simulink model "motionsystem_control_simulation"  (R2017a)
settings: Solver=FixedStepAuto  StartTime=0.0  StopTime=30  FixedStep=dt  RelTol=1e-3
values from neighbouring files (symbols this model uses):
  dt = 0.567    [SimulinkMotionPlot.m]    (also in f.m = 0.001; fJacobian.m = 0.001; h.m = 0.001; hJacobian.m = 0.001)
  K = lqr(A,B,Q_LQR, R_LQR)    [initialize_controller_motionsystem.m]
  Ki = KI(:,1:Ni)    [initialize_controller_motionsystem.m]
  p_init = [2.6192; 0; 2.24]    [initialize_controller_motionsystem.m]
  p_t_init = zeros(3,1)    [initialize_controller_motionsystem.m]
  phi_init = [phix_init; phiy_init]    [initialize_controller_motionsystem.m]
  Pt_init = [-2.395; 3.811; -3.255]    [initialize_controller_motionsystem.m]
libraries: sharedTrackingLibrary x1
settings Model: Creator=Jan  LastModifiedBy=Jan

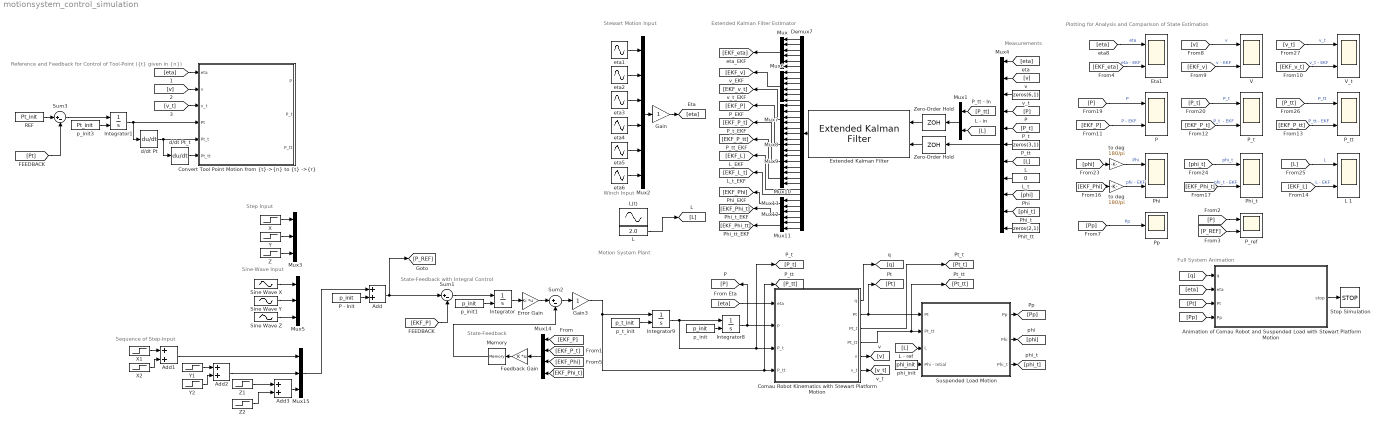
== system motionsystem_control_simulation ==
  note: Step Input
  note: Sine-Wave Input
  note: Sequence of Step-Input
  note: Motion System Plant
  note: Measurements
  note: State-Feedback
  note: Extended Kalman Filter Estimator
  note: Winch Input
  note: Full System Animation
  note: Stewart Motion Input
  note: Plotting for Analysis and Comparison of State Estimation
  note: State-Feedback with Integral Control
  note: Reference and Feedback for Control of Tool-Point
      | ({t} given in {n})
  " L_t " : Constant  Value=0
  " P_tt " : Constant  Value=zeros(3,1)
  " Phit_tt " : Constant  Value=zeros(2,1)
  " Zero-Order Hold " : ZeroOrderHold  SampleTime=dt
  " v_t " : Constant  Value=zeros(6,1)
  Add{,1..3} (4 alike) : Sum
  Animation of Comau Robot and Suspended Load with Stewart Platform Motion : MATLAB Function  TreatAsAtomicUnit=on  SystemSampleTime=0.1
  Comau Robot Kinematics with Stewart Platform Motion : Subsystem
  "Convert Tool Point Motion from {t}->{n} to {t} ->{r}" : MATLAB Function  TreatAsAtomicUnit=on
  Demux7 : Demux  Outputs=35
  Error Gain : Gain  Gain=Ki  Multiplication=Matrix(K*u)
  Eta1 : Scope  NumInputPorts=2
  Extended Kalman Filter : sharedTrackingLibrary/Extended Kalman Filter  StateTransitionFcn=f  HasStateTransitionJacobianFcn=on  StateTransitionJacobianFcn=fJacobian  HasAdditiveProcessNoise=Additive  ProcessNoise=Q_EKF  HasTimeVaryingProcessNoise=off  HasStateTransitionFcnExtraArgument=1  InitialState=EKF_init  InitialStateCovariance=P_EKF  MeasurementFcn1=h  HasMeasurementJacobianFcn1=on  MeasurementJacobianFcn1=hJacobian  HasMeasurementEnablePort1=off  HasAdditiveMeasurementNoise1=Additive  MeasurementNoise1=R_EKF  HasTimeVaryingMeasurementNoise1=off  HasMeasurementFcnExtraArgument1=0  MeasurementFcn2=myMeasurementFcn  HasMeasurementJacobianFcn2=off  HasMeasurementEnablePort2=off  HasAdditiveMeasurementNoise2=Additive  MeasurementNoise2=1  HasTimeVaryingMeasurementNoise2=off  HasMeasurementFcnExtraArgument2=0  MeasurementFcn3=myMeasurementFcn  HasMeasurementJacobianFcn3=off  HasMeasurementEnablePort3=off  HasAdditiveMeasurementNoise3=Additive  MeasurementNoise3=1  HasTimeVaryingMeasurementNoise3=off  HasMeasurementFcnExtraArgument3=0  MeasurementFcn4=myMeasurementFcn  HasMeasurementJacobianFcn4=off  HasMeasurementEnablePort4=off  HasAdditiveMeasurementNoise4=Additive  MeasurementNoise4=1  HasTimeVaryingMeasurementNoise4=off  HasMeasurementFcnExtraArgument4=0  MeasurementFcn5=myMeasurementFcn  HasMeasurementJacobianFcn5=off  HasMeasurementEnablePort5=off  HasAdditiveMeasurementNoise5=Additive  MeasurementNoise5=1  HasTimeVaryingMeasurementNoise5=off  HasMeasurementFcnExtraArgument5=0  EnableMultirate=off  StateTransitionFcnSampleTime=1  MeasurementFcn1SampleTime=1  MeasurementFcn2SampleTime=1  MeasurementFcn3SampleTime=1  MeasurementFcn4SampleTime=1  MeasurementFcn5SampleTime=1  UseCurrentEstimator=on  OutputStateCovariance=off  DataType=double  SampleTime=dt  NumberOfMeasurements=1
  Feedback Gain : Gain  Gain=K  Multiplication=Matrix(K*u)
  Gain : Gain
  Gain3 : Gain
  Integrator{,1,8..9} (4 alike) : Integrator  InitialConditionSource=external
  L : Constant  Value=2.0
  L 1 : Scope  NumInputPorts=2
  L(t) : Sin  Amplitude=0.75  Bias=2.0  Frequency=2*pi*0.05  SampleTime=0
  Memory : Memory
  Mux{,2,6..7} (4 alike) : Mux  Inputs=6
  Mux{1,11..13} (4 alike) : Mux  Inputs=2
  Mux{3,5,8..10,15} (6 alike) : Mux  Inputs=3
  Mux14 : Mux
  Mux4 : Mux  Inputs=11
  P : Scope  NumInputPorts=2
  P - Init : Constant  Value=p_init
  P_ref : Scope  NumInputPorts=2
  P_t : Scope  NumInputPorts=2
  P_tt : Scope  NumInputPorts=2
  Phi : Scope  NumInputPorts=2
  Phi_t : Scope  NumInputPorts=2
  "Pp   " : Scope
  REF : Constant  Value=Pt_init
  Sine Wave X : Sin  Amplitude=0.5  Frequency=2*pi*0.07  SampleTime=0
  Sine Wave Y : Sin  Amplitude=0.3  Frequency=2*pi*0.09  SampleTime=0
  Sine Wave Z : Sin  Amplitude=0.25  Frequency=2*pi*0.15  SampleTime=0
  Stop Simulation : Stop
  Sum1 : Sum  Inputs=|+-
  Sum2 : Sum  Inputs=|+-
  Sum3 : Sum  Inputs=|+-
  Suspended Load Motion : Subsystem
  V : Scope  NumInputPorts=2
  V_t : Scope  NumInputPorts=2
  X : Step  Time=0  After=0.4  SampleTime=0
  X1 : Step  After=0.4  SampleTime=0
  X2 : Step  Time=10  After=-0.8  SampleTime=0
  Y : Step  Time=0  After=0.4  SampleTime=0
  Y1 : Step  Time=2  After=0.4  SampleTime=0
  Y2 : Step  Time=13  After=-0.8  SampleTime=0
  Z : Step  Time=0  After=0.4  SampleTime=0
  Z1 : Step  Time=3  After=0.4  SampleTime=0
  Z2 : Step  Time=9  After=-0.2  SampleTime=0
  "Zero-Order Hold " : ZeroOrderHold  SampleTime=dt
  d/dt Pt : Derivative
  d/dt Pt_t : Derivative
  eta1 : Sin  Amplitude=0.1  Frequency=2*pi*0.1  Phase=0/180*pi  SampleTime=0
  eta2 : Sin  Amplitude=0.1  Frequency=2*pi*0.2  Phase=45/180*pi  SampleTime=0
  eta3 : Sin  Amplitude=0.2  Frequency=2*pi*0.1  Phase=90/180*pi  SampleTime=0
  eta4 : Sin  Amplitude=5/180*pi  Frequency=2*pi*0.1  Phase=0/180*pi  SampleTime=0
  eta5 : Sin  Amplitude=5/180*pi  Frequency=2*pi*0.15  Phase=90/180*pi  SampleTime=0
  eta6 : Sin  Amplitude=5/180*pi  Frequency=2*pi*0.2  Phase=120/180*pi  SampleTime=0
  "p_init " : Constant  Value=p_init
  p_init1 : Constant  Value=p_init
  p_init3 : Constant  Value=Pt_init
  p_t_init : Constant  Value=p_t_init
  phi_init : Constant  Value=phi_init
  to deg : Gain  Gain=180/pi
  "to deg    " : Gain  Gain=180/pi
  wires:
  Comau Robot Kinematics with Stewart Platform Motion/4(Pt_tt) -> [Pt_tt], Suspended Load Motion/2(Pt_tt)
  eta2/1 -> Mux2/2
  Mux2/1 -> Gain/1
  eta3/1 -> Mux2/3
  phi_init/1 -> Suspended Load Motion/4(Phi - Intial)
  eta1/1 -> Mux2/1
  eta6/1 -> Mux2/6
  eta5/1 -> Mux2/5
  Comau Robot Kinematics with Stewart Platform Motion/2(Pt) -> [Pt], Suspended Load Motion/1(Pt)
  eta4/1 -> Mux2/4
  Gain/1 -> [eta]
  Integrator8/1 -> [P], Comau Robot Kinematics with Stewart Platform Motion/2(P)
  "p_init "/1 -> Integrator8/2
  p_t_init/1 -> Integrator9/2
  Comau Robot Kinematics with Stewart Platform Motion/3(Pt_t) -> [Pt_t]
  Suspended Load Motion/3(Phi_t) -> [phi_t]
  Suspended Load Motion/2(Phi) -> [phi]
  Comau Robot Kinematics with Stewart Platform Motion/5(v) -> [v]
  Comau Robot Kinematics with Stewart Platform Motion/6(v_t) -> [v_t]
  Sum1/1 -> Integrator/1
  [EKF_P] -> Sum1/2
  Integrator/1 -> Error Gain/1
  Error Gain/1 -> Sum2/1
  Sum2/1 -> Gain3/1
  [P_tt] -> Mux1/1
  " Phit_tt "/1 -> Mux4/11
  Demux7/16 -> Mux7/4
  Demux7/14 -> Mux7/2
  Mux1/1 -> "Zero-Order Hold "/1
  [eta] -> Mux4/1
  Demux7/3 -> Mux/3
  Demux7/1 -> Mux/1
  [v] -> Mux4/2
  [L] -> Mux4/7
  Demux7/9 -> Mux6/3
  Demux7/4 -> Mux/4
  Demux7/13 -> Mux7/1
  Demux7/34 -> Mux11/1
  Demux7/19 -> Mux8/1
  Demux7/2 -> Mux/2
  Mux9/1 -> [EKF_P_t]
  Demux7/28 -> [EKF_L]
  [P] -> Mux4/4
  Mux13/1 -> [EKF_Phi]
  " P_tt "/1 -> Mux4/6
  Demux7/21 -> Mux8/3
  [P_t] -> Mux4/5
  Demux7/30 -> Mux13/1
  Demux7/22 -> Mux9/1
  " Zero-Order Hold "/1 -> Extended Kalman Filter/2
  Demux7/12 -> Mux6/6
  Demux7/29 -> [EKF_L_t]
  Demux7/32 -> Mux12/1
  [phi_t] -> Mux4/10
  Demux7/31 -> Mux13/2
  Demux7/25 -> Mux10/1
  Mux12/1 -> [EKF_Phi_t]
  Demux7/8 -> Mux6/2
  Demux7/15 -> Mux7/3
  Demux7/24 -> Mux9/3
  Mux7/1 -> [EKF_v_t]
  Mux11/1 -> [EKF_Phi_tt]
  Demux7/33 -> Mux12/2
  " L_t "/1 -> Mux4/8
  Demux7/35 -> Mux11/2
  Extended Kalman Filter/1 -> Demux7/1
  Mux10/1 -> [EKF_P_tt]
  Demux7/11 -> Mux6/5
  Mux/1 -> [EKF_eta]
  Demux7/5 -> Mux/5
  [phi] -> Mux4/9
  Demux7/27 -> Mux10/3
  Mux6/1 -> [EKF_v]
  Demux7/10 -> Mux6/4
  Demux7/18 -> Mux7/6
  Demux7/6 -> Mux/6
  Demux7/17 -> Mux7/5
  " v_t "/1 -> Mux4/3
  Demux7/7 -> Mux6/1
  Demux7/26 -> Mux10/2
  Mux8/1 -> [EKF_P]
  "Zero-Order Hold "/1 -> Extended Kalman Filter/1
  Demux7/20 -> Mux8/2
  Demux7/23 -> Mux9/2
  [v] -> V/1  "v"
  [P_t] -> P_t/1  "P_t"
  to deg/1 -> Phi/2  "phi - EKF"
  "to deg    "/1 -> Phi/1  "Phi"
  [v_t] -> V_t/1  "v_t"
  [phi] -> "to deg    "/1
  [L] -> L 1/1  "L"
  [EKF_L] -> L 1/2  "L - EKF"
  [EKF_Phi_t] -> Phi_t/2  "phi_t - EKF"
  [EKF_P_tt] -> P_tt/2  "P_tt - EKF"
  [phi_t] -> Phi_t/1  "phi_t"
  [EKF_P_t] -> P_t/2  "P_t  - EKF"
  [EKF_v_t] -> V_t/2  "v_t - EKF"
  [EKF_v] -> V/2  "v - EKF"
  [EKF_eta] -> Eta1/2  "eta - EKF"
  [eta] -> Eta1/1  "eta"
  [P_tt] -> P_tt/1  "P_tt"
  [P] -> P/1  "P"
  [EKF_Phi] -> to deg/1
  [EKF_P] -> P/2  "P - EKF"
  Memory/1 -> Sum2/2
  [EKF_Phi_t] -> Mux14/4
  [EKF_P_t] -> Mux14/2
  Feedback Gain/1 -> Memory/1
  [EKF_P] -> Mux14/1
  Mux14/1 -> Feedback Gain/1
  Add/1 -> [P_REF], Sum1/1
  Animation of Comau Robot and Suspended Load with Stewart Platform Motion/1(stop) -> Stop Simulation/1
  Comau Robot Kinematics with Stewart Platform Motion/1(q) -> [q]
  [q] -> Animation of Comau Robot and Suspended Load with Stewart Platform Motion/1(q)
  [Pt] -> Animation of Comau Robot and Suspended Load with Stewart Platform Motion/3(Pt)
  [Pp] -> Animation of Comau Robot and Suspended Load with Stewart Platform Motion/4(Pp)
  [eta] -> Animation of Comau Robot and Suspended Load with Stewart Platform Motion/2(eta)
  Suspended Load Motion/1(Pp) -> [Pp]
  p_init1/1 -> Integrator/2
  p_init3/1 -> Integrator1/2
  REF/1 -> Sum3/1
  [Pt] -> Sum3/2
  Sum3/1 -> Integrator1/1
  Integrator1/1 -> d/dt Pt/1, "Convert Tool Point Motion from {t}->{n} to {t} ->{r}"/4(Pt)
  d/dt Pt/1 -> "Convert Tool Point Motion from {t}->{n} to {t} ->{r}"/5(Pt_t), d/dt Pt_t/1
  d/dt Pt_t/1 -> "Convert Tool Point Motion from {t}->{n} to {t} ->{r}"/6(Pt_tt)
  [eta] -> "Convert Tool Point Motion from {t}->{n} to {t} ->{r}"/1(eta)
  [v] -> "Convert Tool Point Motion from {t}->{n} to {t} ->{r}"/2(v)
  [v_t] -> "Convert Tool Point Motion from {t}->{n} to {t} ->{r}"/3(v_t)
  Mux4/1 -> " Zero-Order Hold "/1
  [Pp] -> "Pp   "/1  "Pp"
  [eta] -> Comau Robot Kinematics with Stewart Platform Motion/1(eta)
  [L] -> Suspended Load Motion/3(L)
  [L] -> Mux1/2
  [EKF_Phi] -> Mux14/3
  X/1 -> Mux3/1
  Y/1 -> Mux3/2
  Z/1 -> Mux3/3
  P - Init/1 -> Add/2
  Sine Wave X/1 -> Mux5/1
  Sine Wave Y/1 -> Mux5/2
  Sine Wave Z/1 -> Mux5/3
  [P] -> P_ref/1
  [P_REF] -> P_ref/2
  Z1/1 -> Add3/1
  Add2/1 -> Mux15/2
  Add1/1 -> Mux15/1
  X1/1 -> Add1/1
  X2/1 -> Add1/2
  Y1/1 -> Add2/1
  Y2/1 -> Add2/2
  Add3/1 -> Mux15/3
  Z2/1 -> Add3/2
  Gain3/1 -> Integrator9/1, [P_tt], Comau Robot Kinematics with Stewart Platform Motion/4(P_tt)
  Integrator9/1 -> Integrator8/1, [P_t], Comau Robot Kinematics with Stewart Platform Motion/3(P_t)
  Mux15/1 -> Add/1
  L/1 -> [L]

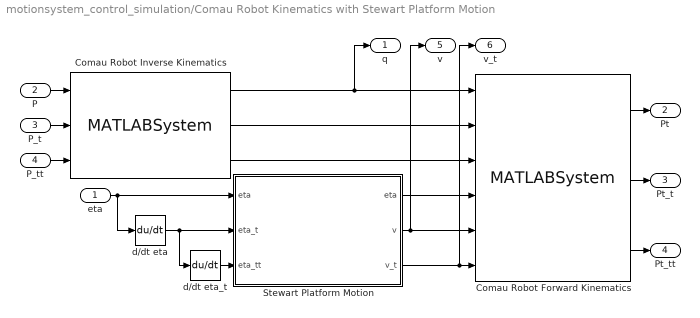
== system motionsystem_control_simulation/Comau Robot Kinematics with Stewart Platform Motion ==
  eta : Inport
  P : Inport  Port=2
  P_t : Inport  Port=3
  P_tt : Inport  Port=4
  Comau Robot Forward Kinematics : MATLABSystem  System=ComauRobotSystem  StringChoice=Stewart Motion  SimulateUsing=Code generation
      mask Type: ComauRobotSystem
      mask Display:
      | disp('ComauRobotSystem');
      | port_label('input',1,'q');
      | port_label('input',2,'q_t');
      | port_label('input',3,'q_tt');
      | port_label('input',4,'eta');
      | port_label('input',5,'v');
      | port_label('input',6,'v_t');
      | port_label('output',1,'Pt');
      | port_label('output',2,'Pt_t');
      | port_label('output',3,'Pt_tt');
  Comau Robot Inverse Kinematics : MATLABSystem  System=ComauRobotSystem  StringChoice=Inverse Kinematics  SimulateUsing=Code generation
      mask Type: ComauRobotSystem
      mask Display:
      | disp('ComauRobotSystem');
      | port_label('input',1,'P');
      | port_label('input',2,'P_t');
      | port_label('input',3,'P_tt');
      | port_label('output',1,'q');
      | port_label('output',2,'q_t');
      | port_label('output',3,'q_tt');
  Stewart Platform Motion : MATLAB Function  TreatAsAtomicUnit=on
  d/dt eta : Derivative
  d/dt eta_t : Derivative
  q : Outport
  Pt : Outport  Port=2
  Pt_t : Outport  Port=3
  Pt_tt : Outport  Port=4
  v : Outport  Port=5
  v_t : Outport  Port=6
  wires:
  d/dt eta/1 -> Stewart Platform Motion/2(eta_t), d/dt eta_t/1
  Comau Robot Forward Kinematics/2 -> Pt_t/1
  Comau Robot Forward Kinematics/3 -> Pt_tt/1
  Stewart Platform Motion/1(eta) -> Comau Robot Forward Kinematics/4
  Stewart Platform Motion/3(v_t) -> v_t/1, Comau Robot Forward Kinematics/6
  Stewart Platform Motion/2(v) -> Comau Robot Forward Kinematics/5, v/1
  d/dt eta_t/1 -> Stewart Platform Motion/3(eta_tt)
  Comau Robot Forward Kinematics/1 -> Pt/1
  eta/1 -> Stewart Platform Motion/1("eta "), d/dt eta/1
  P/1 -> Comau Robot Inverse Kinematics/1
  P_t/1 -> Comau Robot Inverse Kinematics/2
  P_tt/1 -> Comau Robot Inverse Kinematics/3
  Comau Robot Inverse Kinematics/1 -> Comau Robot Forward Kinematics/1, q/1
  Comau Robot Inverse Kinematics/2 -> Comau Robot Forward Kinematics/2
  Comau Robot Inverse Kinematics/3 -> Comau Robot Forward Kinematics/3

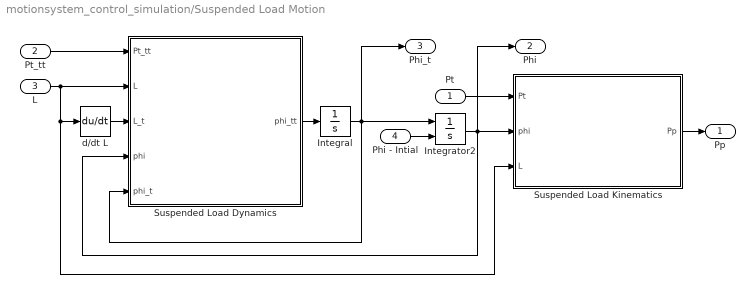
== system motionsystem_control_simulation/Suspended Load Motion ==
  Pt : Inport
  Pt_tt : Inport  Port=2
  L : Inport  Port=3
  Phi - Intial : Inport  Port=4
  Integral : Integrator  InitialCondition=[0 0]
  Integrator2 : Integrator  InitialConditionSource=external
  Suspended Load Dynamics : MATLAB Function  TreatAsAtomicUnit=on
  Suspended Load Kinematics : MATLAB Function  TreatAsAtomicUnit=on
  d/dt L : Derivative
  Pp : Outport
  Phi : Outport  Port=2
  Phi_t : Outport  Port=3
  wires:
  Pt/1 -> Suspended Load Kinematics/1(Pt)
  Suspended Load Dynamics/1(phi_tt) -> Integral/1
  Pt_tt/1 -> Suspended Load Dynamics/1(Pt_tt)
  L/1 -> Suspended Load Kinematics/3(L), d/dt L/1, Suspended Load Dynamics/2(L)
  Integral/1 -> Phi_t/1, Integrator2/1, Suspended Load Dynamics/5(phi_t)
  Integrator2/1 -> Phi/1, Suspended Load Kinematics/2(phi), Suspended Load Dynamics/4(phi)
  Phi - Intial/1 -> Integrator2/2
  Suspended Load Kinematics/1(Pp) -> Pp/1
  d/dt L/1 -> Suspended Load Dynamics/3(L_t)

== matlab function motionsystem_control_simulation/Suspended Load Motion/Suspended Load Dynamics ==
  data: Pt_tt input; L input; L_t input; phi_tt output; phi input; phi_t input
function phi_tt = pendulumDynamics(Pt_tt, L, L_t, phi, phi_t)
    % Calculates the dynamics of the suspended load
    % Derives the differential equation for the euler angles
    %
    % Input: 
    %	Pt_tt   : Tool-point acceleration
    %	phi     : Pendulum Angular position euler angles
    %   phit_t  : Pendulum Angular velocity euler angles
    %   L       : Wire length
    %   L_t     : Wire velocity
    %
    %   Output  :
    %   phit_t  : Pendulum Angular acceleration euler angles
    
    % Parameters
    g = 9.81;   % Gravity
    
    % Tool-point acceleration components
    xt_tt = Pt_tt(1); 
    yt_tt = Pt_tt(2); 
    zt_tt = Pt_tt(3);

    % Pendulum euler angles (angular position)
    phix = phi(1);
    phiy = phi(2);

    % Pendulum euler angles (angular velocity)
    phix_t = phi_t(1);
    phiy_t = phi_t(2);
    
     % Pendulum ODE of the euler angles
    % (found from euler-lagrange equation,
    %  derived by the use of Maple)
    phix_tt = (xt_tt*cos(phix) + yt_tt*sin(phix)*sin(phiy) ...
              - zt_tt*sin(phix)*cos(phiy) ...
              - g*sin(phix)*cos(phiy) ...
              - 2*L_t*phix_t ...
              - L*phiy_t^2*sin(phix)*cos(phix)) / L;

    phiy_tt = (- yt_tt*cos(phiy) - zt_tt*sin(phiy) ...
              - g*sin(phiy) + 2*L_t*phiy_t*cos(phix) ...
              + 2*L*phix_t*phiy_t*sin(phix)) ...
              / (L*cos(phix));

    phi_tt = [phix_tt; phiy_tt];

== matlab function motionsystem_control_simulation/Convert Tool Point Motion from {t}->{n} to {t} ->{r} ==
  data: eta input; P output; v input; v_t input; Pt input; Pt_t input; Pt_tt input; P_t output; P_tt output
function [P, P_t, P_tt] = toolPointConvertion(eta, v, v_t, Pt, Pt_t, Pt_tt)
    % Transformation matrix found from calibration
    % Robot pose relative to motion frame of Stewart Platform
    % {b} -> {r}
    Hbr = [-0.4972,	0.8676,	-0.0050,	-1.0820;    
            0.8676,	0.4972,	 0.0012,     1.5360;
            0.0036,-0.0037, -1.0000,	-1.0245;
                 0,      0,       0,     1.0000];  
            
    % Body fixed velocity and acceleration skew matrices
    Sw = math3d.Skew(v(4:6));
    Sw_t = math3d.Skew(v_t(4:6));
            
    % Ship/Stewart relative to static csys {n} -> {b}
    Rnb = math3d.Rzyx(eta(4:6));
    Rnb_t = Rnb*Sw;
    Rnb_tt = Rnb*Sw*Sw + Rnb*Sw_t;
            
    % Constant offset between stewart platform and robot base
    % {b} -> {r}
    r = Hbr(1:3,4);
    Rbr = Hbr(1:3,1:3);
    
    % Tool-point position relative to Robot Base
    % {t}/{r} given in {r}
    P = inv(Rbr)*(inv(Rnb)*(Pt - eta(1:3)) - r);
    
    % Tool-point velocity relative to Robot Base
    % {t}/{r} given in {r}
    P_t = inv(Rbr)*(inv(Rnb)*(Pt_t - v(1:3) - Rnb_t*(r + Rbr*P)));
    
    % Tool-point acceleration relative to Robot Base
    % {t}/{r} given in {r}
    P_tt = inv(Rbr)*(inv(Rnb)*(Pt_tt - v_t(1:3) - Rnb_tt*(r + Rbr*P) ...
                               - 2*Rnb_t*(Rbr*P_t)));

== matlab function motionsystem_control_simulation/Suspended Load Motion/Suspended Load Kinematics ==
  data: Pt input; phi input; L input; Pp output
function Pp = pendulumKinematics(Pt, phi, L)
    % Calculates the kinematics of the suspended load
    
    % Input: 
    %	Pt_tt   : Tool-point position
    %	phi     : Pendulum Angular position euler angles
    %   L       : Wire length
    
%     % Load in calibration structure
%     motionlab = load('calib.mat');
% 
%     % Transformation matrices found from calibration 
%     Hgn = motionlab.calib.WORLD_TO_EM8000.H; 
    
    % Tool-point position 
    xt = Pt(1);
    yt = Pt(2);
    zt = Pt(3);

    % Pendulum euler angles
    phix = phi(1);
    phiy = phi(2);

    % Pendulum position 
    xp = xt - L*sin(phix);
    yp = yt + L*cos(phix)*sin(phiy);
    zp = zt + L*cos(phix)*cos(phiy);

    Pp = [xp; yp; zp];
    
%     Pp = Hgn*[Pp; 1];
%     Pp = Pp(1:3);
end

== matlab function motionsystem_control_simulation/Comau Robot Kinematics with Stewart Platform Motion/Stewart Platform Motion ==
  data: eta input; eta output; eta_t input; eta_tt input; v output; v_t output
function [eta, v, v_t] = stewartMotion(eta, eta_t, eta_tt)
    % Calculate the relative Velocity and Acceleration component 
    % of the Stewart platform
    %
    % Input: 
    %	eta     : Orientation of {b} -> {n}
    %	eta_t   : Velocity of {b} -> {n}
    %   eta_tt	: Acceleration of {b} -> {n}
    %
    % Output:
    %   eta     : Orientation of {b} -> {n}
    %   v       : Body fixed velocity {n}/{b} given in {b}
    %   v_t      : Body fixed acceleration {n}/{b} given in {b}
    
% s : Angle Sequence
% ('zyx' is used for simulation)
% ('xyz' is used when motion data is obtained from MRU)
s = 'zyx';

% Velocity
J = vJacobian(eta, s);
v = J\eta_t;

% Acceleration
J_t = aJacobian(eta, eta_t, s);
v_t = J\(eta_tt - J_t*v);

end

function J = vJacobian(eta, s)
    phi = eta(4);
    theta = eta(5);
    psi = eta(6);

    if strcmp(s, 'xyz')
        T11 = cos(psi)/cos(theta);
        T12 = -sin(psi)/cos(theta);
        T13 = 0;
        
        T21 = sin(psi);
        T22 = cos(psi);
        T23 = 0;
        
        T31 = -(cos(psi)*sin(theta))/cos(theta);
        T32 = (sin(psi)*sin(theta))/cos(theta);
        T33 = 1;
        
        T = [T11,	T12,	T13;
             T21,   T22,    T23;
             T31,   T32,    T33];
         
        J = [eye(3), zeros(3);
             zeros(3), T];
        
    elseif strcmp(s, 'zyx')
        T11 = 1;
        T12 = (sin(phi)*sin(theta))/cos(theta);
        T13 = (cos(phi)*sin(theta))/cos(theta);
        
        T21 = 0;
        T22 = cos(phi);
        T23 = -sin(phi);
        
        T31 = 0;
        T32 = sin(phi)/cos(theta);
        T33 = cos(phi)/cos(theta);
        
        T = [T11,	T12,	T13;
             T21,   T22,    T23;
             T31,   T32,    T33];
         
        J = [eye(3), zeros(3);
             zeros(3), T];
    end
end

function J_t = aJacobian(eta, eta_t, s)
    phi = eta(4);
    theta = eta(5);
    psi = eta(6);
    
    phi_t = eta_t(4);
    theta_t = eta_t(5);
    psi_t = eta_t(6);

    if strcmp(s, 'xyz')
        
        T11 = (cos(psi)*sin(theta)*theta_t ...
               - cos(theta)*sin(psi)*psi_t)/cos(theta)^2;
        T12 = -(cos(theta)*cos(psi)*psi_t ...
              + sin(theta)*sin(psi)*theta_t)/cos(theta)^2;
        T13 = 0;
        
        T21 = cos(psi)*psi_t;
        T22 = -sin(psi)*psi_t;
        T23 = 0;
        
        T31 = -(cos(psi)*theta_t ...
              - cos(theta)*sin(theta)*sin(psi)*psi_t)/cos(theta)^2;
        T32 = (sin(psi)*theta_t ...
             + cos(theta)*cos(psi)*sin(theta)*psi_t)/cos(theta)^2;
        T33 = 0;
        
        T = [T11,	T12,	T13;
             T21,   T22,    T23;
             T31,   T32,    T33];
         
        J_t = [zeros(3), zeros(3);
               zeros(3), T];
        
    elseif strcmp(s, 'zyx')
      
        T11 = 0;
        T12 = (sin(phi)*theta_t ...
            + cos(phi)*cos(theta)*sin(theta)*phi_t)/cos(theta)^2;
        T13 = (cos(phi)*theta_t ...
            - cos(theta)*sin(phi)*sin(theta)*phi_t)/cos(theta)^2;
        
        T21 = 0;
        T22 = -sin(phi)*phi_t;
        T23 = -cos(phi)*phi_t;
        
        T31 = 0;
        T32 = (cos(phi)*cos(theta)*phi_t ...
            + sin(phi)*sin(theta)*theta_t)/cos(theta)^2;
        T33 = -(cos(theta)*sin(phi)*phi_t ...
            - cos(phi)*sin(theta)*theta_t)/cos(theta)^2;
        T = [T11,	T12,	T13;
             T21,   T22,    T23;
             T31,   T32,    T33];
         
        J_t = [zeros(3), zeros(3);
               zeros(3), T];
    end
end

== matlab function motionsystem_control_simulation/Animation of Comau Robot and Suspended Load with Stewart Platform Motion ==
  data: q input; eta input; stop output; Pt input; Pp input
function stop = SimulinkMotionPlot(q, eta, Pt, Pp)
    % Creates a 3D-animation for the motion of the motion-lab system
    % Requires values for the Comau Robot joints and stewart platform
    % Input: 
    %	q	: Robot joint angular position
    %   eta	: Stewart platform orientation
    %	Pt	: Tool-point position
    %	phi	: Pendulum Angular position euler angles
    % Output:
    %	stop :  Bool value to stop the anitmation
    
    % Persistent variables, to only be initialized once
    persistent h;           % Plot
    persistent motionlab;   % Calibration structure
    % Transformation matrices
    persistent Hgn;         % World to EM8000  {g} -> {n}
    persistent Hbr;         % EM8000 to Comau  {b} -> {r}
    persistent Hg;          % World coordinate system (Reference CSYS)
    
    stop = false;
    
    %% Initialization 
    % One time intitialization of plotting settings
    if isempty(h)
        % Close previous all plots
        close all
        
        % Plotting setup
        h = figure('Name','Motion Lab Animation');
        
        xlabel('x-axis')
        ylabel('y-axis')
        zlabel('z-axis')
        xlim([-5, 3])
        ylim([-3, 5])
        zlim([0, 8])
        
        hold on;
        grid on;
        view(-30,20);
        
        % Load in calibration structure
        motionlab = load('calib.mat');
        
        % Transformation matrices found from calibration 
        Hgn = motionlab.calib.WORLD_TO_EM8000.H;  % {g} -> {n}
        Hbr = motionlab.calib.EM8000_TO_COMAU.H;  % {b} -> {r}
        
        % Reference coordinate system (world coordinate)
        Hg = eye(4);
    end
    
    %% Drawing
    if ishandle(h)
        cla;
        
        % Plot the motion of the Stewart Platform
        Hgb = plot_stewartplatformpose(eta, Hg, Hgn);
        
        % Tranformation from World CSYS to Robot Base
        Hgr = Hgb*Hbr;
        
        % Plot Robot pose relative to input CSYS
        plot_robotpose(q, Hgr);
        
        % Plot Pendulum pose relative to input CSYS
        plot_pendulum(Pt, Pp, Hgn);
        
        drawnow;
    end
    
    %% Destructor
    if ~ishandle(h)
        stop = true;
    end
    
end

%% Child functions

% Plot the pose of the stewart platform
% This includes the reference world coordinate
function Hgb = plot_stewartplatformpose(eta, Hg, Hgn)
    % Input:
    %   eta     : Stewart platform orientation
    %   Hg      : World coordinate system (Reference CSYS)
    %   Hgn     : Transformation matrix, World to EM8000 {g} -> {n}
    % Output:
    %   Hgb     : Transformation matrix, World to EM8000 {g} -> {b}
    
    % Motion from intial platform pose to motion
    % {n} -> {b}
    Hnb = eye(4);
    Hnb(1:3,1:3) = math3d.Rzyx(eta(4:6));	% Rotation matrix
    Hnb(1:3,4) = eta(1:3);                  % Translation vector

    % Relative transformation
    Hgb = Hgn*Hnb;  % World to EM8000 (motion) {g} -> {b}

    % Plot coordinate system
    plot_coordinatesystem(Hg);      % Reference
    plot_coordinatesystem(Hgn);     % EM8000 static
    plot_coordinatesystem(Hgb);     % EM8000 motion
end

% Plot the pose of the Comau Robot
% This includes links and local coordinate systems
function plot_robotpose(q, Hr)
    % Inputs:
    % Hr : Transformation matrix of the robot base [4x4]
    % q  : Robot joints [3x1]
    
    % Static link lengths
    a1 = 0.350;
    a2 = 1.160;
    a3 = 0.250;
    d1 = 0.830;
    d4 = 1.4922;
    d6 = 0.210;
    dt = 0.567;
    L = d4 + d6 + dt;
    
    % Joint angles
    q1 = q(1);
    q2 = q(2);
    q3 = q(3);

    % Robot DH Table
    T1 = math3d.DH(-q1, d1, a1, pi/2);
    T2 = math3d.DH(pi/2 - q2, 0, a2, 0);
    T3 = math3d.DH(q3 + pi/2 + q2, 0, a3, pi/2);
    T4 = math3d.DH(pi, L, 0, 0);
            
    % Relative transformation
    Hr1 = Hr*T1;   % Robot base to joint q1 {r -> q1}
    Hr2 = Hr1*T2;   % Robot base to joint q2 {r -> q2}
    Hr3 = Hr2*T3;   % Robot base to joint q3 {r -> q2}
    Hr4 = Hr3*T4;   % Robot base to tool-point {r -> t}
    
    % Plot coordinate systems
    plot_coordinatesystem(Hr);      % Base
    plot_coordinatesystem(Hr1);     % Joint q1
    plot_coordinatesystem(Hr2);     % Joint q2
    plot_coordinatesystem(Hr3);     % Joint q3
    plot_coordinatesystem(Hr4);     % Tool-Point

    % Plot links
    plot_line(Hr(1:3,4), Hr1(1:3,4));	% Base to joint q1        
    plot_line(Hr1(1:3,4), Hr2(1:3,4));	% joint q1 to joint q2 
    plot_line(Hr2(1:3,4), Hr3(1:3,4));	% joint q2 to joint q3 
    plot_line(Hr3(1:3,4), Hr4(1:3,4));	% joint q3 to Tool-point
    
end

% Plot the position of the Pendulum
function plot_pendulum(Pt, Pp, Hr)
    % Inputs:
    % Pt    :   Tool-point position [3x]
    % Pp    :   Pendulum position [3x1]
    % Hr    :   Transformation matrix of the robot base [4x4]
    
    % Transforming the Position vector relative to world CSYS
    Pt = Hr*[Pt; 1];
    Pp = Hr*[Pp; 1];
    
    % Correction of Z-direction
    L = 2.0;    % Initial Wire length
    Pp(3) = Pp(3);
    
    % Pendulum positions
    xp = Pp(1);
    yp = Pp(2);
    zp = Pp(3);
    
    % Plot wire
    plot_line(Pt(1:3), Pp(1:3));

    % Plot Load
    plot3(xp, yp, zp, 'ro', 'LineWidth', 5);
end
        
% Plot a line in 3D plots
function plot_line(p1, p2)
    % Inputs:
    %   p1  :   Point 1 [x1; y1; z1]
    %   p2  :   Point 2 [x2; y2; z2]

    % Pre-allocate
    line = zeros(2,3);

    line(1,:) = p1;
    line(2,:) = p2;

    X = line(:,1);
    Y = line(:,2);
    Z = line(:,3);

    plot3(X, Y, Z, 'k', 'LineWidth', 1)
end
        
% Plot the coordinate system in 3D plots
% with default rgb-colors to the related axis.
function plot_coordinatesystem(H)
    % Inputs:
    %   H       :   Transformation-matrix (size = 4x4)

    % Pre-allocate
    axis = zeros(2,3);
    
    % Rotation and Translation
    d = H(1:3,4);   % Translation vector
    R = H(1:3,1:3); % Rotation matrix

    % Axis colors
    colors = {'r', 'g', 'b'};
    
    % Length of each axis in csys
    csys_len = 0.5;
    
    % Plot all 3 axis
    % (Looping through plotting one axis at a time)
    for i = 1:3
        axis(1,:) = d;                      % csys origo [x0 y0 z0]
        axis(2,:) = d + R(:,i)*csys_len;    % end point of axis [x y z]

        X = axis(:,1);  % Vector of the x-component
        Y = axis(:,2);  % Vector of the y-component
        Z = axis(:,3);  % Vector of the z-component

        % Plot one of the axis with the related color
        plot3(X, Y, Z, colors{i}, 'LineWidth', 1)
    end
end
